simulink model "main"  (R2022b)
settings: Solver=FixedStepDiscrete  StartTime=0.0  StopTime=30  FixedStep=0.005  RelTol=1e-3
libraries: simulink x1
settings Model: DataDictionary=main.sldd  PauseTimes=4  ExtModeTrigDuration=2  Creator=F64236C  LastModifiedBy=F64236C
settings OptimizationCC: EnhancedBackFolding=on  PassReuseOutputArgsAs=Individual arguments  ZeroExternalMemoryAtStartup=off  ZeroInternalMemoryAtStartup=off  MaxStackSize=64  OptimizeBlockOrder=speed  DifferentSizesBufferReuse=on  OptimizationCustomize=off  EfficientTunableParamExpr=on
settings DebuggingCC: ParameterTunabilityLossMsg=error
settings HardwareCC: ProdBitPerPointer=32  ProdBitPerSizeT=32  ProdBitPerPtrDiffT=32  ProdLargestAtomicInteger=Long  ProdLargestAtomicFloat=Double  ProdWordSize=32  ProdHWDeviceType=ARM Compatible->ARM Cortex
settings SFSimCC: MATLABDynamicMemAlloc=off
settings RTWCC: Description=Embedded Coder  SystemTargetFile=ert.tlc  HardwareBoard=ESP32-WROOM(Arduino Compatible)  TLCOptions="-aInlineSetEventsForThisBaseRateFcn=TLC_FALSE -aSuppressMultiTaskScheduler=TLC_FALSE  -aRateBasedStepFcn=0"  TemplateMakefile=ert_default_tmf  Toolchain=ESP32  BuildConfiguration=Faster Runs
settings CodeAppCC: ForceParamTrailComments=on  IgnoreCustomStorageClasses=off  OperatorAnnotations=on  SimulinkDataObjDesc=on  SFDataObjDesc=on  InsertBlockDesc=on
settings ERTTargetCC: TargetLangStandard=C99 (ISO)  SupportContinuousTime=on  SupportNonInlinedSFcns=on  SupportVariableSizeSignals=on  ExtModeTransport=3  ExtModeStaticAlloc=on  ExtModeAutomaticAllocSize=off  ExtModeStaticAllocSize=65536  ExtModeMexFile=ext_xcp  ExtModeIntrfLevel=Level2 - Open  RootIOFormat=Structure reference

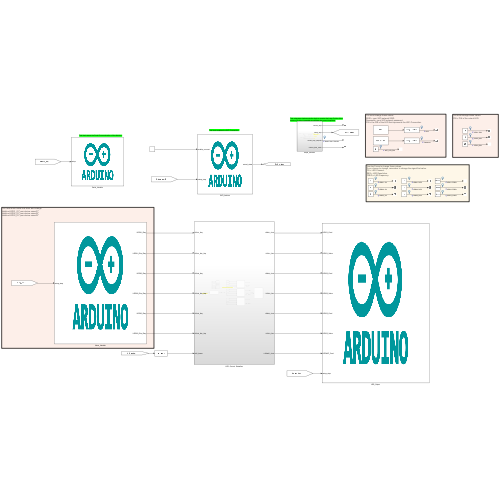
[thumbnail: Simulink's stored preview of the top-level diagram]
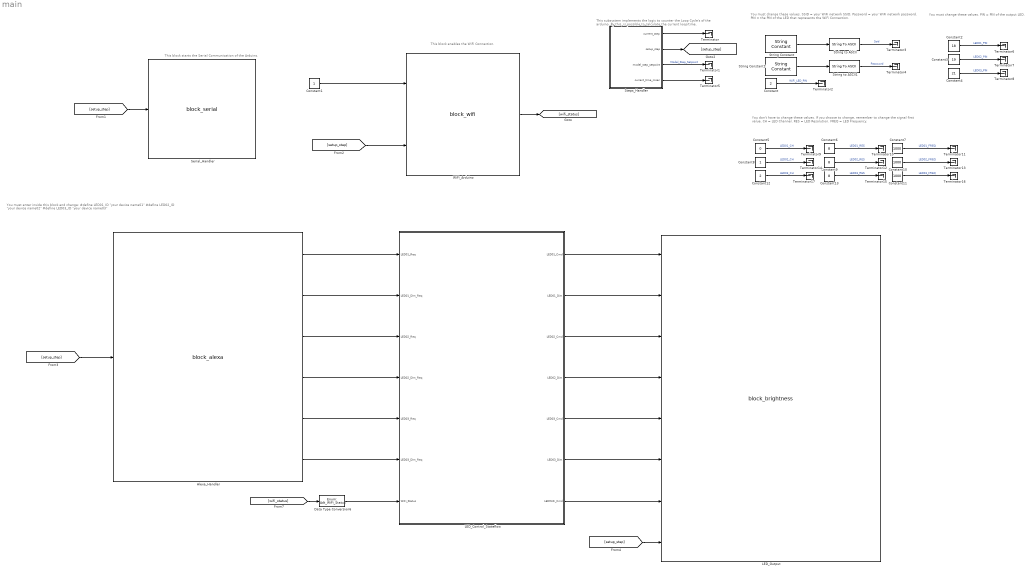
== system main ==
  note: You must enter inside this block and change:
      | #define LED01_ID "your device name01"
      | #define LED02_ID "your device name02"
      | #define LED03_ID "your device name03"
  note: You must change these values.
      | SSID = your WiFi network SSID.
      | Password = your WiFi network password.
      | PIN = the PIN of the LED that represents the WiFi Connection.
  note: You must change these values.
      | PIN = PIN of the output LED.
  note: You don't have to change these values.
      | If you choose to change, remember to change the signal first value.
      | CH = LED Channel.
      | RES = LED Resolution.
      | FREQ = LED Frequency.
  note: This block enables the WiFi Connection.
  note: This block starts the Serial Communication of the Arduino.
  note: This subsystem implements the logic to counter the Loop Cycle's of the arduino. By this, is possible to calculate the current loop/time.
  Alexa_Handler : S-Function  Priority=4  FunctionName=block_alexa  SFunctionModules=block_alexa_wrapper.cpp  SFunctionDeploymentMode=off  EnableBusSupport=off  mask(S-Function Builder){}
      mask help: Simulink:masks:SFunctionBuilder_MD
      mask init:
      | val = [[.9  0.75 0.75 1 1 .9 .9 1]',[1 1 0.75 0.75 .9 .9 1 .9]'];try , sys = get_param(gcb,'SfunBuilderFcnName');if isempty(sys), sys = get_param(gcb,'FunctionName'); end,catch, sys = get_param(gcb,'FunctionName'); end
      settings: CopyFcn=set_param(gcbh,'LinkStatus','none')  OpenFcn=sfunctionwizard(gcbh)
      mask Display:
      | image('../imgs/arduino_logo.png');
      | port_label('input',1,'setup_step')
      | port_label('output',1,'LED01_Req')
      | port_label('output',2,'LED01_Dim_Req')
      | port_label('output',3,'LED02_Req')
      | port_label('output',4,'LED02_Dim_Req')
      | port_label('output',5,'LED03_Req')
      | port_label('output',6,'LED03_Dim_Req')
  Constant : Constant  Value=2  OutDataTypeStr=uint8
  Constant1 : Constant  OutDataTypeStr=boolean
  Constant10 : Constant  Value=1000  OutDataTypeStr=uint16
  Constant11 : Constant  Value=1000  OutDataTypeStr=uint16
  Constant12 : Constant  Value=2  OutDataTypeStr=uint8
  Constant13 : Constant  Value=8  OutDataTypeStr=uint8
  Constant2 : Constant  Value=18  OutDataTypeStr=uint8
  Constant3 : Constant  Value=19  OutDataTypeStr=uint8
  Constant4 : Constant  Value=21  OutDataTypeStr=uint8
  Constant5 : Constant  Value=0  OutDataTypeStr=uint8
  Constant6 : Constant  Value=8  OutDataTypeStr=uint8
  Constant7 : Constant  Value=1000  OutDataTypeStr=uint16
  Constant8 : Constant  OutDataTypeStr=uint8
  Constant9 : Constant  Value=8  OutDataTypeStr=uint8
  Data Type Conversion6 : DataTypeConversion  OutDataTypeStr=Enum: Adt_WiFi_Status  SaturateOnIntegerOverflow=off  RndMeth=Floor
  LED_Control_Stateflow : Subsystem
  LED_Output : S-Function  FunctionName=block_brightness  SFunctionModules=block_brightness_wrapper.cpp  SFunctionDeploymentMode=off  EnableBusSupport=off  mask(S-Function Builder){}
      mask help: Simulink:masks:SFunctionBuilder_MD
      mask init: same as main/Alexa_Handler
      settings: CopyFcn=set_param(gcbh,'LinkStatus','none')  OpenFcn=sfunctionwizard(gcbh)
      mask Display:
      | image('../imgs/arduino_logo.png');
      | port_label('input',1,'LED01_Cmd')
      | port_label('input',2,'LED01_Value')
      | port_label('input',3,'LED02_Cmd')
      | port_label('input',4,'LED02_Value')
      | port_label('input',5,'LED03_Cmd')
      | port_label('input',6,'LED03_Value')
      | port_label('input',7,'LEDWiFi_Cmd')
      | port_label('input',8,'setup_step')
  Serial_Handler : S-Function  Priority=1  FunctionName=block_serial  SFunctionModules=block_serial_wrapper.cpp  SFunctionDeploymentMode=off  EnableBusSupport=off  mask(S-Function Builder){}
      mask help: Simulink:masks:SFunctionBuilder_MD
      mask init: same as main/Alexa_Handler
      settings: CopyFcn=set_param(gcbh,'LinkStatus','none')  OpenFcn=sfunctionwizard(gcbh)
      mask Display:
      | image('../imgs/arduino_logo.png');
      | 
      | port_label('input',1,'setup')
  Steps_Handler : Subsystem
  String Constant : StringConstant  String="\"ssid\""
  String Constant1 : StringConstant  String="\"password\""
  String to ASCII : StringToASCII  OutputVectorSize=32
  String to ASCII1 : StringToASCII  OutputVectorSize=32
  Terminator{,1..17} (18 alike) : Terminator
  WiFi_Arduino : S-Function  Priority=2  FunctionName=block_wifi  SFunctionModules=block_wifi_wrapper.cpp  SFunctionDeploymentMode=off  EnableBusSupport=off  mask(S-Function Builder){}
      mask help: Simulink:masks:SFunctionBuilder_MD
      mask init: same as main/Alexa_Handler
      settings: CopyFcn=set_param(gcbh,'LinkStatus','none')  OpenFcn=sfunctionwizard(gcbh)
      mask Display:
      | image('../imgs/arduino_logo.png');
      | port_label('input',1,'enable_connect')
      | port_label('input',2,'setup_step')
      | port_label('output',1,'actual_state')
  wires:
  WiFi_Arduino/1 -> [wifi_status]
  String to ASCII1/1 -> Terminator4/1  "Password"
  String Constant1/1 -> String to ASCII1/1
  String to ASCII/1 -> Terminator3/1  "Ssid"
  String Constant/1 -> String to ASCII/1
  Steps_Handler/1(current_step) -> Terminator/1
  Steps_Handler/4(current_time_msec) -> Terminator5/1
  Steps_Handler/3(model_step_setpoint) -> Terminator1/1  "Model_Step_Setpoint"
  [setup_step] -> Serial_Handler/1
  Steps_Handler/2(setup_step) -> [setup_step]
  [setup_step] -> WiFi_Arduino/2
  Constant1/1 -> WiFi_Arduino/1
  Constant/1 -> Terminator2/1  "WiFi_LED_PIN"
  Constant2/1 -> Terminator6/1  "LED01_PIN"
  Constant3/1 -> Terminator7/1  "LED02_PIN"
  Constant4/1 -> Terminator8/1  "LED03_PIN"
  Constant5/1 -> Terminator9/1  "LED01_CH"
  Constant6/1 -> Terminator10/1  "LED01_RES"
  Constant7/1 -> Terminator11/1  "LED01_FREQ"
  Constant10/1 -> Terminator13/1  "LED02_FREQ"
  Constant9/1 -> Terminator12/1  "LED02_RES"
  Constant8/1 -> Terminator14/1  "LED02_CH"
  Constant11/1 -> Terminator16/1  "LED03_FREQ"
  Constant12/1 -> Terminator17/1  "LED03_CH"
  Constant13/1 -> Terminator15/1  "LED03_RES"
  [wifi_status] -> Data Type Conversion6/1
  Data Type Conversion6/1 -> LED_Control_Stateflow/7(WiFi_Status)
  LED_Control_Stateflow/1(LED01_Cmd) -> LED_Output/1
  LED_Control_Stateflow/2(LED01_Dim) -> LED_Output/2
  LED_Control_Stateflow/7(LEDWiFi_Cmd) -> LED_Output/7
  [setup_step] -> LED_Output/8
  LED_Control_Stateflow/3(LED02_Cmd) -> LED_Output/3
  LED_Control_Stateflow/4(LED02_Dim) -> LED_Output/4
  LED_Control_Stateflow/5(LED03_Cmd) -> LED_Output/5
  LED_Control_Stateflow/6(LED03_Dim) -> LED_Output/6
  Alexa_Handler/4 -> LED_Control_Stateflow/4(LED02_Dim_Req)
  Alexa_Handler/3 -> LED_Control_Stateflow/3(LED02_Req)
  Alexa_Handler/5 -> LED_Control_Stateflow/5(LED03_Req)
  Alexa_Handler/2 -> LED_Control_Stateflow/2(LED01_Dim_Req)
  Alexa_Handler/6 -> LED_Control_Stateflow/6(LED03_Dim_Req)
  Alexa_Handler/1 -> LED_Control_Stateflow/1(LED01_Req)
  [setup_step] -> Alexa_Handler/1

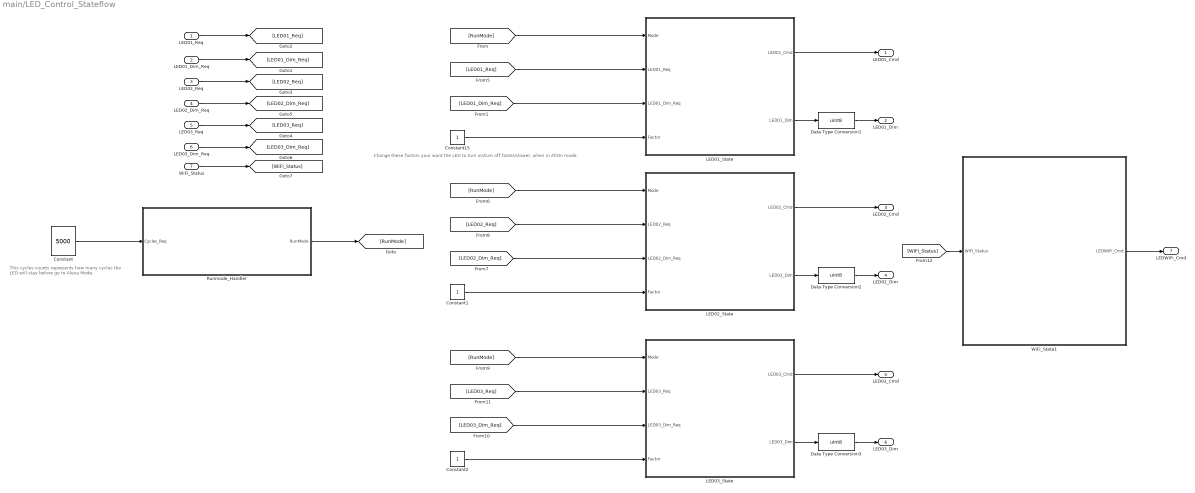
== system main/LED_Control_Stateflow ==
  note: Change these factors your want the LED to turn on/turn off faster/slower, when in AllOn mode.
  note: This cycles counts represents how many cycles the LED will stay before go to Alexa Mode.
  LED01_Req : Inport
  LED01_Dim_Req : Inport  Port=2
  LED02_Req : Inport  Port=3
  LED02_Dim_Req : Inport  Port=4
  LED03_Req : Inport  Port=5
  LED03_Dim_Req : Inport  Port=6
  WiFi_Status : Inport  Port=7
  Constant : Constant  Value=5000  OutDataTypeStr=uint16
  Constant1 : Constant  OutDataTypeStr=double
  Constant15 : Constant  OutDataTypeStr=double
  Constant2 : Constant  OutDataTypeStr=double
  Data Type Conversion1 : DataTypeConversion  OutDataTypeStr=uint8  SaturateOnIntegerOverflow=off  RndMeth=Floor
  Data Type Conversion2 : DataTypeConversion  OutDataTypeStr=uint8  SaturateOnIntegerOverflow=off  RndMeth=Floor
  Data Type Conversion3 : DataTypeConversion  OutDataTypeStr=uint8  SaturateOnIntegerOverflow=off  RndMeth=Floor
  LED01_State : Stateflow chart  TreatAsAtomicUnit=on
  LED02_State : Stateflow chart  TreatAsAtomicUnit=on
  LED03_State : Stateflow chart  TreatAsAtomicUnit=on
  Runmode_Handler : Stateflow chart  TreatAsAtomicUnit=on
  WiFi_State1 : Stateflow chart  TreatAsAtomicUnit=on
  LED01_Cmd : Outport
  LED01_Dim : Outport  Port=2
  LED02_Cmd : Outport  Port=3
  LED02_Dim : Outport  Port=4
  LED03_Cmd : Outport  Port=5
  LED03_Dim : Outport  Port=6
  LEDWiFi_Cmd : Outport  Port=7
  wires:
  Constant15/1 -> LED01_State/4(Factor)
  LED01_State/2(LED01_Dim) -> Data Type Conversion1/1
  LED01_State/1(LED01_Cmd) -> LED01_Cmd/1
  Data Type Conversion1/1 -> LED01_Dim/1
  [RunMode] -> LED01_State/1(Mode)
  LED01_Dim_Req/1 -> [LED01_Dim_Req]
  [LED01_Dim_Req] -> LED01_State/3(LED01_Dim_Req)
  LED01_Req/1 -> [LED01_Req]
  LED02_Req/1 -> [LED02_Req]
  LED03_Req/1 -> [LED03_Req]
  LED02_Dim_Req/1 -> [LED02_Dim_Req]
  LED03_Dim_Req/1 -> [LED03_Dim_Req]
  [LED01_Req] -> LED01_State/2(LED01_Req)
  Data Type Conversion2/1 -> LED02_Dim/1
  [LED02_Req] -> LED02_State/2(LED02_Req)
  LED02_State/1(LED02_Cmd) -> LED02_Cmd/1
  Constant1/1 -> LED02_State/4(Factor)
  LED02_State/2(LED02_Dim) -> Data Type Conversion2/1
  [LED02_Dim_Req] -> LED02_State/3(LED02_Dim_Req)
  [RunMode] -> LED02_State/1(Mode)
  Constant2/1 -> LED03_State/4(Factor)
  Data Type Conversion3/1 -> LED03_Dim/1
  LED03_State/1(LED03_Cmd) -> LED03_Cmd/1
  [LED03_Dim_Req] -> LED03_State/3(LED03_Dim_Req)
  [RunMode] -> LED03_State/1(Mode)
  LED03_State/2(LED03_Dim) -> Data Type Conversion3/1
  [LED03_Req] -> LED03_State/2(LED03_Req)
  WiFi_Status/1 -> [WiFi_Status]
  [WiFi_Status] -> WiFi_State1/1(WiFi_Status)
  WiFi_State1/1(LEDWiFi_Cmd) -> LEDWiFi_Cmd/1
  Runmode_Handler/1(RunMode) -> [RunMode]
  Constant/1 -> Runmode_Handler/1(Cycles_Req)

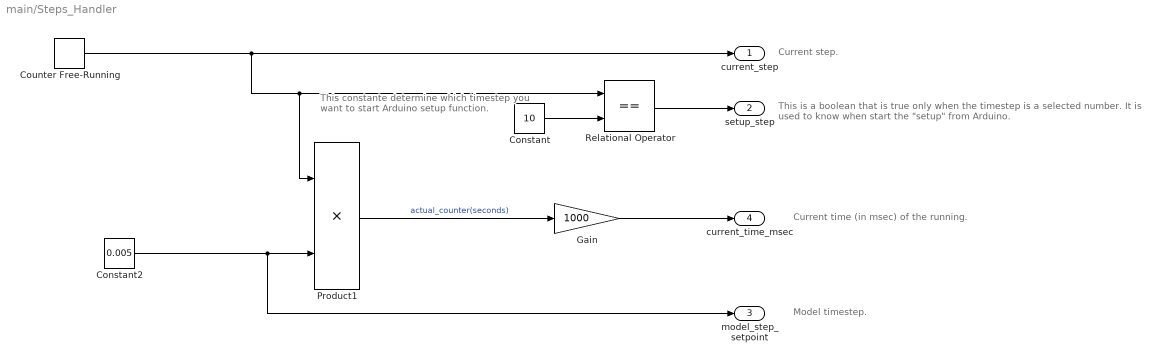
== system main/Steps_Handler ==
  note: This constante determine which timestep you want to start Arduino setup function.
  note: This is a boolean that is true only when the timestep is a selected number.
      | It is used to know when start the "setup" from Arduino.
  note: Model timestep.
  note: Current time (in msec) of the running.
  note: Current step.
  Constant : Constant  Value=10
  Constant2 : Constant  Value=0.005  OutDataTypeStr=double
  Counter Free-Running : simulink/Sources/Counter Free-Running  NumBits=32  tsamp=-1
  Gain : Gain  Gain=1000
  Product1 : Product  OutDataTypeStr=double
  Relational Operator : RelationalOperator  Operator===  OutDataTypeStr=boolean  RndMeth=Simplest  InputSameDT=off
  current_step : Outport  OutDataTypeStr=uint32
  setup_step : Outport  Port=2
  model_step_setpoint : Outport  Port=3  OutDataTypeStr=double
  current_time_msec : Outport  Port=4  OutDataTypeStr=double
  wires:
  Constant2/1 -> model_step_setpoint/1, Product1/2
  Counter Free-Running/1 -> Product1/1, Relational Operator/1, current_step/1
  Product1/1 -> Gain/1  "actual_counter(seconds)"
  Constant/1 -> Relational Operator/2
  Relational Operator/1 -> setup_step/1
  Gain/1 -> current_time_msec/1

== stateflow chart main/LED_Control_Stateflow/LED03_State ==
  state DIM_DecreaseFcn [function]
    (default) -> (junction 12)
    (junction 12) -> (junction 13) : {LED03_Dim = LED03_Dim - Factor;}
  state DIM_IncreaseFcn [function]
    (default) -> (junction 17)
    (junction 17) -> (junction 18) : {LED03_Dim = LED03_Dim + Factor;}
  state MODE
    en:
    LED03_Cmd = LED03_Req;
    LED03_Dim = LED03_Dim_Req;
    du:
    LED03_Cmd = LED03_Req;
    LED03_Dim = LED03_Dim_Req;
  state INCREMENT
    en:
    LED03_Dim = 1;
    du:
    DIM_IncreaseFcn();
    LED03_Cmd = true;
  state DECREMENT
    en:
    LED03_Dim = 255;
    du:
    DIM_DecreaseFcn();
    LED03_Cmd = true;
  (default) -> MODE [order 1]
  MODE -> INCREMENT : [Mode == Adt_RunMode.AllOn]
  (default) -> MODE [order 2] : [Mode ~= Adt_RunMode.AllOn]
  DECREMENT -> MODE [order 2] : [Mode ~= Adt_RunMode.AllOn]
  DECREMENT -> INCREMENT [order 1] : [LED03_Dim <= 2 && Mode == Adt_RunMode.AllOn]
  INCREMENT -> DECREMENT : [LED03_Dim >= 254 && Mode == Adt_RunMode.AllOn]
  data: Mode input Enum: Adt_RunMode; LED03_Req input boolean; LED03_Dim_Req input double; LED03_Cmd output boolean; LED03_Dim output double; Factor input double

== stateflow chart main/LED_Control_Stateflow/WiFi_State1 ==
  state WiFi_LED [function]
    (default) -> (junction 4)
    (junction 4) -> (junction 5) [order 1] : [WiFi_Status==Adt_WiFi_Status.Connected]
    (junction 4) -> (junction 7) [order 2]
    (junction 5) -> (junction 6) : {LEDWiFi_Cmd=true}
    (junction 7) -> (junction 6) : {LEDWiFi_Cmd=false}
  state Start
    du:
    WiFi_LED();
  (default) -> Start
  data: LEDWiFi_Cmd output boolean; WiFi_Status input Enum: Adt_WiFi_Status

== stateflow chart main/LED_Control_Stateflow/LED02_State ==
  state DIM_IncreaseFcn [function]
    (default) -> (junction 17)
    (junction 17) -> (junction 18) : {LED02_Dim = LED02_Dim + Factor;}
  state DIM_DecreaseFcn [function]
    (default) -> (junction 12)
    (junction 12) -> (junction 13) : {LED02_Dim = LED02_Dim - Factor;}
  state MODE
    en:
    LED02_Cmd = LED02_Req;
    LED02_Dim = LED02_Dim_Req;
    du:
    LED02_Cmd = LED02_Req;
    LED02_Dim = LED02_Dim_Req;
  state INCREMENT
    en:
    LED02_Dim = 1;
    du:
    DIM_IncreaseFcn();
    LED02_Cmd = true;
  state DECREMENT
    en:
    LED02_Dim = 255;
    du:
    DIM_DecreaseFcn();
    LED02_Cmd = true;
  (default) -> MODE [order 1]
  MODE -> INCREMENT : [Mode == Adt_RunMode.AllOn]
  (default) -> MODE [order 2] : [Mode ~= Adt_RunMode.AllOn]
  DECREMENT -> MODE [order 2] : [Mode ~= Adt_RunMode.AllOn]
  DECREMENT -> INCREMENT [order 1] : [LED02_Dim <= 2 && Mode == Adt_RunMode.AllOn]
  INCREMENT -> DECREMENT : [LED02_Dim >= 254 && Mode == Adt_RunMode.AllOn]
  data: Mode input Enum: Adt_RunMode; LED02_Req input boolean; LED02_Dim_Req input double; LED02_Cmd output boolean; LED02_Dim output double; Factor input double

== stateflow chart main/LED_Control_Stateflow/Runmode_Handler ==
  state CyclesCount [function]
    (default) -> (junction 12)
    (junction 12) -> (junction 18) [order 1] : [Count >= Cycles_Req]
    (junction 12) -> (junction 14) [order 2] : [Count < Cycles_Req]
    (junction 18) -> (junction 17) : {JobDone = true;}
    (junction 14) -> (junction 17) : {JobDone = false;}
  state Out
    en:
    JobDone = false;
    du:
    Count = Count + uint16(1);
    RunMode = Adt_RunMode.AllOn;
    CyclesCount();
  state In
    en:
    %JobDone = false;
    du:
    Count = uint16(0);
    RunMode = Adt_RunMode.Alexa;
  (default) -> Out
  In -> Out : [JobDone  == false]
  Out -> In : [JobDone == true]
  data: RunMode output Enum: Adt_RunMode; Count local uint16 =uint16(0); Cycles_Req input uint16; JobDone local boolean

== stateflow chart main/LED_Control_Stateflow/LED01_State ==
  state DIM01_IncreaseFcn [function]
    (default) -> (junction 17)
    (junction 17) -> (junction 18) : {LED01_Dim = LED01_Dim + Factor;}
  state DIM01_DecreaseFcn [function]
    (default) -> (junction 12)
    (junction 12) -> (junction 13) : {LED01_Dim = LED01_Dim - Factor;}
  state MODE
    en:
    LED01_Cmd = LED01_Req;
    LED01_Dim = LED01_Dim_Req;
    du:
    LED01_Cmd = LED01_Req;
    LED01_Dim = LED01_Dim_Req;
  state INCREMENT
    en:
    LED01_Dim = 1;
    du:
    DIM01_IncreaseFcn();
    LED01_Cmd = true;
  state DECREMENT
    en:
    LED01_Dim = 255;
    du:
    DIM01_DecreaseFcn();
    LED01_Cmd = true;
  (default) -> MODE [order 1]
  MODE -> INCREMENT : [Mode == Adt_RunMode.AllOn]
  (default) -> MODE [order 2] : [Mode ~= Adt_RunMode.AllOn]
  DECREMENT -> MODE [order 2] : [Mode ~= Adt_RunMode.AllOn]
  DECREMENT -> INCREMENT [order 1] : [LED01_Dim <= 2 && Mode == Adt_RunMode.AllOn]
  INCREMENT -> DECREMENT : [LED01_Dim >= 254 && Mode == Adt_RunMode.AllOn]
  data: Mode input Enum: Adt_RunMode; LED01_Req input boolean; LED01_Dim_Req input double; LED01_Cmd output boolean; LED01_Dim output double; Factor input double
